simulink model "FSM"  (R2023a)
settings: Solver=FixedStepDiscrete  StartTime=0.0  StopTime=10.0  FixedStep=0.1  RelTol=1e-3  EnableMultiTasking=on
settings Model: Creator=sanbaosu  LastModifiedBy=sanbaosu
settings SolverCC: AlgebraicLoopSolver=TrustRegion  AutoInsertRateTranBlk=on
settings DataIOCC: LimitDataPoints=on
settings OptimizationCC: LifeSpan=inf
settings DebuggingCC: UnconnectedInputMsg=warning  UnconnectedOutputMsg=warning  UnconnectedLineMsg=warning  AllowSymbolicDim=off  SFUnexpectedBacktrackingDiag=warning  SFNoUnconditionalDefaultTransitionDiag=warning  SFExecutionAtInitializationDiag=none  ArithmeticOperatorsInVariantConditions=warning
settings ModelReferenceCC: EnableRefExpFcnMdlSchedulingChecks=on
settings SFSimCC: SimUseLocalCustomCode=off  CustomCodeUndefinedFunction=UseInterfaceOnly
settings RTWCC: RTWUseLocalCustomCode=off  DLArmComputeVersion=19.05
settings CodeAppCC: StateflowObjectComments=on
settings GRTTargetCC: TargetLangStandard=C89/C90 (ANSI)
settings ConfigComp: CovMetricSettings=dw  CovSaveCumulativeToWorkspaceVar=on  CovSaveSingleToWorkspaceVar=on  CovExternalEMLEnable=off  CovSFcnEnable=off

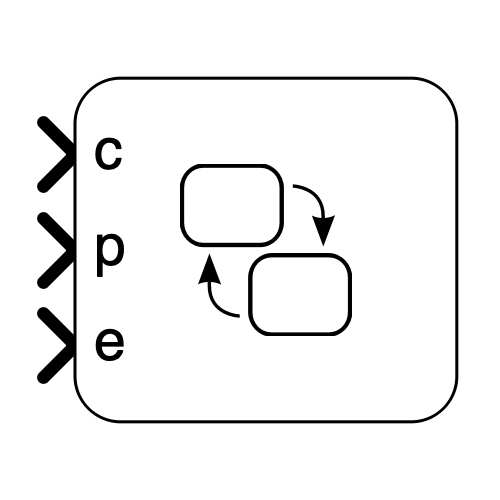
[thumbnail: Simulink's stored preview of the top-level diagram]
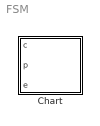
== system FSM ==
  Chart : Stateflow chart  TreatAsAtomicUnit=on

== stateflow chart FSM/Chart ==
  state L
  state R
  state ACC
  state BL
  state BR
  L -> (junction 23)
  (junction 27) -> L [order 1] : [c == 1, e == 1]
  (junction 19) -> L [order 2] : [c == 1, e == 1]
  (junction 19) -> R [order 1] : [c == -1, e == 1]
  (junction 34) -> R [order 1] : [c == -1, e == 1]
  R -> (junction 31)
  (junction 23) -> ACC [order 2] : [c == 1, p == 1]
  (junction 31) -> ACC [order 2] : [c == -1, p == 1]
  (junction 23) -> BL [order 1] : [c == 1, e == 0]
  (junction 31) -> BR [order 1] : [c == -1, e == 0]
  ACC -> (junction 19)
  (default) -> ACC
  (junction 27) -> ACC [order 2] : [c == 1, p == 0, e == 0]
  (junction 34) -> ACC [order 2] : [c == -1, p == 0, e == 0]
  BL -> (junction 27)
  BR -> (junction 34)
  data: c input; p input; e input
